simulink model "state_feedback_ed"  (Simulink 8.9)
settings: Solver=ode45  StartTime=0.0  StopTime=10.0  RelTol=1e-3
values from neighbouring files (symbols this model uses):
  k = acker(A,B,P)    [state_feedback_and_observer.m]    (also in state_feedback_and_observer2.m)
  L = acker(A',C',P1)    [state_feedback_and_observer.m]    (also in state_feedback_and_observer2.m)
settings Model: Creator=taewon  LastModifiedBy=edward
settings DataIOCC: LimitDataPoints=off  SaveFormat=StructureWithTime  SignalLoggingSaveFormat=Dataset
settings DebuggingCC: UnderspecifiedInitializationDetection=Simplified  MergeDetectMultiDrivingBlocksExec=error  FcnCallInpInsideContextMsg=error  StateNameClashWarn=none  SFUnexpectedBacktrackingDiag=error  SFNoUnconditionalDefaultTransitionDiag=error
settings HardwareCC: ProdBitPerPointer=64  ProdLargestAtomicFloat=Float  ProdIntDivRoundTo=Zero  ProdEndianess=LittleEndian  ProdHWDeviceType=Specified
settings ModelReferenceCC: PropagateSignalLabelsOutOfModel=on
settings GRTTargetCC: GeneratePreprocessorConditionals=Use local settings  CombineOutputUpdateFcns=on  GRTInterface=off
settings ConfigComp: CovMetricSettings=dwe  CovHtmlReporting=off  CovSaveCumulativeToWorkspaceVar=off  CovSaveSingleToWorkspaceVar=off  CovExternalEMLEnable=on

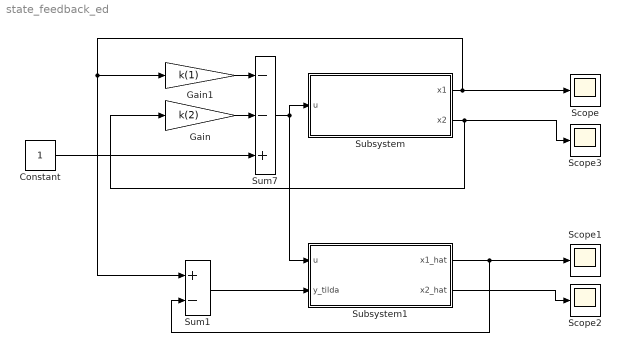
== system state_feedback_ed ==
  Constant : Constant
  Gain : Gain  Gain=k(2)
  Gain1 : Gain  Gain=k(1)
  Scope{,1..3} (4 alike) : Scope
  Subsystem : Subsystem
  Subsystem1 : Subsystem
  Sum1 : Sum  Inputs=+-
  Sum7 : Sum  Inputs=--+
  wires:
  Subsystem/1(x1) -> Sum1/1, Gain1/1, Scope/1
  Subsystem/2(x2) -> Gain/1, Scope3/1
  Gain/1 -> Sum7/2
  Gain1/1 -> Sum7/1
  Sum7/1 -> Subsystem/1(u), Subsystem1/1(u)
  Constant/1 -> Sum7/3
  Sum1/1 -> Subsystem1/2(y_tilda)
  Subsystem1/1(x1_hat) -> Sum1/2, Scope1/1
  Subsystem1/2(x2_hat) -> Scope2/1

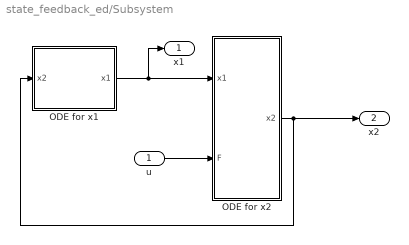
== system state_feedback_ed/Subsystem ==
  u : Inport
  ODE for x1 : Subsystem
  ODE for x2 : Subsystem
  x1 : Outport
  x2 : Outport  Port=2
  wires:
  ODE for x2/1(x2) -> x2/1, ODE for x1/1(x2)
  u/1 -> ODE for x2/2(F)
  ODE for x1/1(x1) -> x1/1, ODE for x2/1(x1)

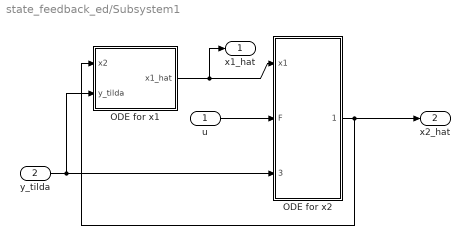
== system state_feedback_ed/Subsystem1 ==
  u : Inport
  y_tilda : Inport  Port=2
  ODE for x1 : Subsystem
  ODE for x2 : Subsystem
  x1_hat : Outport
  x2_hat : Outport  Port=2
  wires:
  ODE for x2/1(x2_hat) -> x2_hat/1, ODE for x1/1(x2)
  u/1 -> ODE for x2/2(F)
  ODE for x1/1(x1_hat) -> x1_hat/1, ODE for x2/1(x1)
  y_tilda/1 -> ODE for x2/3(y_tilda), ODE for x1/2(y_tilda)

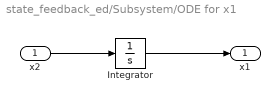
== system state_feedback_ed/Subsystem/ODE for x1 ==
  x2 : Inport
  Integrator : Integrator
  x1 : Outport
  wires:
  x2/1 -> Integrator/1
  Integrator/1 -> x1/1

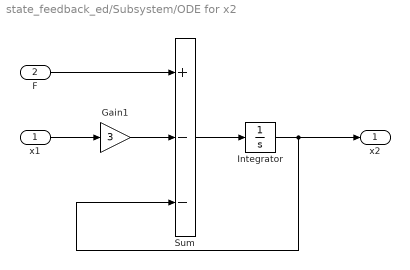
== system state_feedback_ed/Subsystem/ODE for x2 ==
  x1 : Inport
  F : Inport  Port=2
  Gain1 : Gain  Gain=3
  Integrator : Integrator
  Sum : Sum  Inputs=+--
  x2 : Outport
  wires:
  Sum/1 -> Integrator/1
  Integrator/1 -> Sum/3, x2/1
  Gain1/1 -> Sum/2
  x1/1 -> Gain1/1
  F/1 -> Sum/1

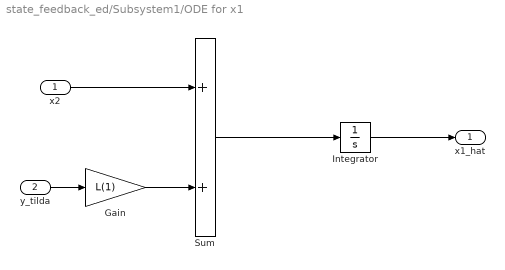
== system state_feedback_ed/Subsystem1/ODE for x1 ==
  x2 : Inport
  y_tilda : Inport  Port=2
  Gain : Gain  Gain=L(1)
  Integrator : Integrator
  Sum : Sum  Inputs=2
  x1_hat : Outport
  wires:
  Integrator/1 -> x1_hat/1
  x2/1 -> Sum/1
  Sum/1 -> Integrator/1
  Gain/1 -> Sum/2
  y_tilda/1 -> Gain/1

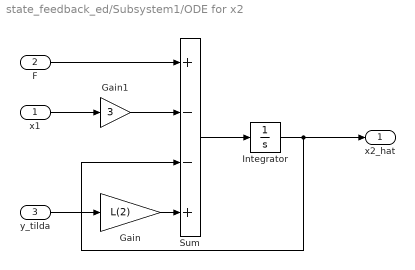
== system state_feedback_ed/Subsystem1/ODE for x2 ==
  x1 : Inport
  F : Inport  Port=2
  y_tilda : Inport  Port=3
  Gain : Gain  Gain=L(2)
  Gain1 : Gain  Gain=3
  Integrator : Integrator
  Sum : Sum  Inputs=+--+
  x2_hat : Outport
  wires:
  Sum/1 -> Integrator/1
  Integrator/1 -> Sum/3, x2_hat/1
  Gain1/1 -> Sum/2
  x1/1 -> Gain1/1
  F/1 -> Sum/1
  Gain/1 -> Sum/4
  y_tilda/1 -> Gain/1
